simulink model "mA2_thruster_as"  (R2023a)
settings: Solver=ode4  StartTime=0.0  StopTime=10.0  FixedStep=0.01  RelTol=1e-3
settings Model: Creator=tobiasvt  LastModifiedBy=HalvorPlatou
settings SolverCC: AlgebraicLoopSolver=TrustRegion
settings DebuggingCC: UnconnectedInputMsg=warning  UnconnectedOutputMsg=warning  UnconnectedLineMsg=warning
settings ModelReferenceCC: EnableRefExpFcnMdlSchedulingChecks=on
settings SFSimCC: CustomCodeUndefinedFunction=UseInterfaceOnly
settings RTWCC: Description=FMU based on GRT (Functional Mock-up Unit)  SystemTargetFile=grtfmi.tlc  GenerateMakefile=off  TemplateMakefile=none  RetainRTWFile=on
settings STFCustomTargetCC: ConcurrentExecutionCompliant=off  CombineOutputUpdateFcns=on  CodeInterfacePackaging=Reusable function  GRTInterface=off  GenerateAllocFcn=on  UseToolchainInfoCompliant=off  SystemTargetFile=grtfmi.tlc
settings GRTTargetCC: ParMdlRefBuildCompliant=off  CompOptLevelCompliant=off  ConcurrentExecutionCompliant=off  MatFileLogging=off  CodeInterfacePackaging=Reusable function  CPPClassGenCompliant=off  GenerateAllocFcn=on  UseToolchainInfoCompliant=off

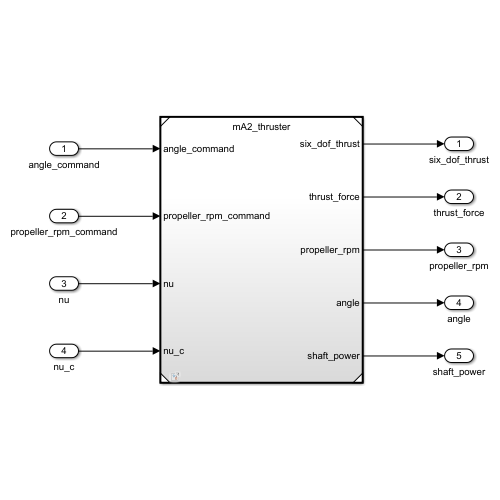
[thumbnail: Simulink's stored preview of the top-level diagram]
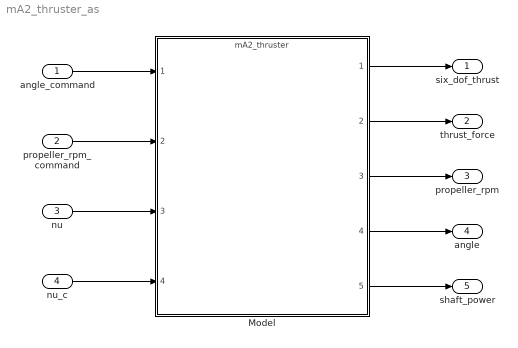
== system mA2_thruster_as ==
  angle_command : Inport
  propeller_rpm_command : Inport  Port=2
  nu : Inport  Port=3  PortDimensions=6
  nu_c : Inport  Port=4  PortDimensions=6
  Model : ModelReference  ModelNameDialog=mA2_thruster.slx  SimulationMode=Normal  ModelReferenceVersion=7.0
  six_dof_thrust : Outport  VectorParamsAs1DForOutWhenUnconnected=off
  thrust_force : Outport  Port=2  VectorParamsAs1DForOutWhenUnconnected=off
  propeller_rpm : Outport  Port=3  VectorParamsAs1DForOutWhenUnconnected=off
  angle : Outport  Port=4  VectorParamsAs1DForOutWhenUnconnected=off
  shaft_power : Outport  Port=5
  wires:
  angle_command/1 -> Model/1
  propeller_rpm_command/1 -> Model/2
  nu/1 -> Model/3
  nu_c/1 -> Model/4
  Model/1 -> six_dof_thrust/1
  Model/2 -> thrust_force/1
  Model/3 -> propeller_rpm/1
  Model/4 -> angle/1
  Model/5 -> shaft_power/1
